simulink model "frictionTest"  (R2014b)
settings: Solver=ode45  StartTime=0.0  StopTime=10.0  RelTol=1e-3
values from neighbouring files (symbols this model uses):
  s = tf('s')    [InitModel.m]    (also in SystemModel.m; SystemModel_marco.m)
undefined symbols (not defined in the file or in its folder): motor
libraries: cstblocks x2, simulink x1
settings Model: Creator=Edoardo  LastModifiedBy=Edoardo

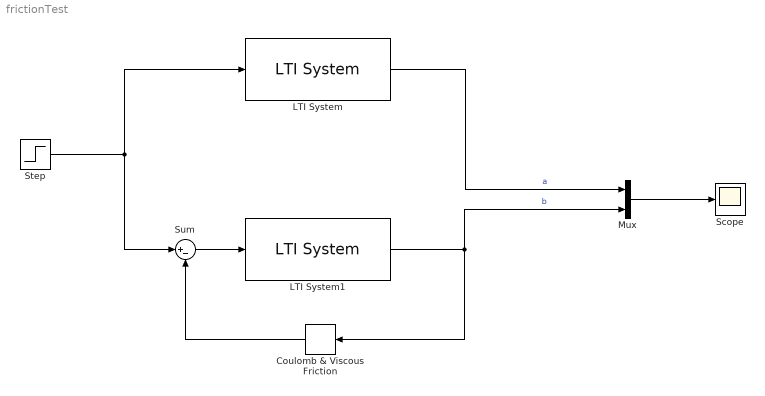
== system frictionTest ==
  Coulomb & Viscous Friction : simulink/Discontinuities/Coulomb & Viscous Friction  offset=motor.coulomb  gain=motor.beta
  LTI System : cstblocks/LTI System  sys=1/(s*motor.J+motor.beta);  IC=[]
  LTI System1 : cstblocks/LTI System  sys=1/(s*motor.J);  IC=[]
  Mux : Mux  Inputs=2
  Scope : Scope
      settings: ShowLegends=on  TimeRange=10
  Step : Step  SampleTime=0
  Sum : Sum  Inputs=|+-
  wires:
  Step/1 -> LTI System/1, Sum/1
  Mux/1 -> Scope/1
  LTI System1/1 -> Mux/2, Coulomb & Viscous Friction/1  "b"
  Sum/1 -> LTI System1/1
  LTI System/1 -> Mux/1  "a"
  Coulomb & Viscous Friction/1 -> Sum/2
